simulink model "mpc_works"  (R2019b)
settings: Solver=VariableStepAuto  StartTime=0.0  StopTime=100  RelTol=1e-3
values from neighbouring files (symbols this model uses):
  Ts = 0.1    [mpcobj1.m]
libraries: simulink x1, mpclib x1
settings Model: PacingRate=0.350000  Creator=deepa  LastModifiedBy=deepa
settings SolverCC: MaxConsecutiveMinStep=100

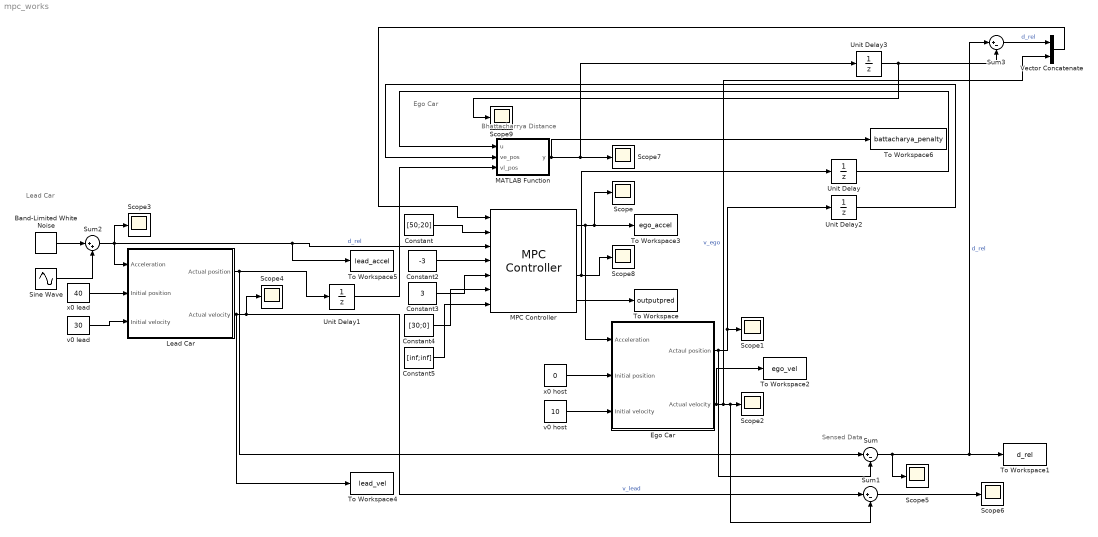
== system mpc_works ==
  note: Bhattacharrya Distance
  note: Lead Car
  note: Sensed Data
  note: Ego Car
  Band-Limited White Noise : simulink/Sources/Band-Limited White Noise  Cov=0.1  Ts=0.1  seed=[23341]
  Constant : Constant  Value=[50;20]
  Constant2 : Constant  Value=-3
  Constant3 : Constant  Value=3
  Constant4 : Constant  Value=[30;0]
  Constant5 : Constant  Value=[inf;inf]
  Ego Car : Subsystem
  Lead Car : Subsystem
  MATLAB Function : MATLAB Function  TreatAsAtomicUnit=on
  MPC Controller : mpclib/MPC Controller  SCDEnableBlockLinearizationSpecification=on  mpcobj=mpcobj  is_multiple=0  enable_value=0  return_u0=off  updateMPCinCallerWorkspace=on  md_inport=on  mv_inport=off  uref_inport=off  return_cost=off  return_mvseq=on  return_qpstatus=off  return_xseq=on  return_state=off  return_ovseq=on  state_inport=off  umin_inport=on  umax_inport=on  ymin_inport=on  ymax_inport=on  cc_inport=off  ywt_inport=off  uwt_inport=off  duwt_inport=off  rhoeps_inport=off  pm_inport=off  MaximumP=10  HorizonChoice=FixedHorizon  n_ts=0.1  n_p=10  n_mv=1  n_md=1  n_ud=0  n_mo=2  n_uo=0  BlockDataType=double  SampleTimeInherited=off  switch_inport=off
  Scope{,1..9} (10 alike) : Scope
  Sine Wave : Sin  Frequency=0.5  SampleTime=Ts
  Sum : Sum  Inputs=|+-
  Sum1 : Sum  Inputs=|+-
  Sum2 : Sum  Inputs=|++
  Sum3 : Sum  Inputs=|+-
  To Workspace : ToWorkspace  VariableName=outputpred  SampleTime=-1
  To Workspace1 : ToWorkspace  VariableName=d_rel  SaveFormat=Timeseries  SampleTime=-1
  To Workspace2 : ToWorkspace  VariableName=ego_vel  SaveFormat=Timeseries  SampleTime=-1
  To Workspace3 : ToWorkspace  VariableName=ego_accel  SaveFormat=Timeseries  SampleTime=-1
  To Workspace4 : ToWorkspace  VariableName=lead_vel  SaveFormat=Timeseries  SampleTime=-1
  To Workspace5 : ToWorkspace  VariableName=lead_accel  SaveFormat=Timeseries  SampleTime=-1
  To Workspace6 : ToWorkspace  VariableName=battacharya_penalty  SaveFormat=Timeseries  SampleTime=-1
  Unit Delay : UnitDelay  InitialCondition=rand(11,4)  SampleTime=-1  HasFrameUpgradeWarning=on
  Unit Delay1 : UnitDelay  SampleTime=-1  HasFrameUpgradeWarning=on
  Unit Delay2 : UnitDelay  SampleTime=-1  HasFrameUpgradeWarning=on
  Unit Delay3 : UnitDelay  SampleTime=-1  HasFrameUpgradeWarning=on
  Vector Concatenate : Concatenate
  v0 host : Constant  Value=10  SampleTime=Ts
  v0 lead : Constant  Value=30  SampleTime=Ts
  x0 host : Constant  Value=0  SampleTime=Ts
  x0 lead : Constant  Value=40  SampleTime=Ts
  wires:
  Sum2/1 -> MPC Controller/3, To Workspace5/1, Scope3/1, Lead Car/1(Acceleration)  "d_rel"
  Lead Car/1(Actual position) -> Unit Delay1/1, Sum/1
  Lead Car/2(Actual velocity) -> Scope4/1, Sum1/1, To Workspace4/1  "v_lead"
  Band-Limited White Noise/1 -> Sum2/1
  v0 lead/1 -> Lead Car/3(Initial velocity)
  x0 lead/1 -> Lead Car/2(Initial position)
  Sum/1 -> Sum3/1, To Workspace1/1, Scope5/1  "d_rel"
  Sum1/1 -> Scope6/1
  MPC Controller/3 -> Unit Delay/1, Scope8/1
  Sine Wave/1 -> Sum2/2
  x0 host/1 -> Ego Car/2(Initial position)
  Constant2/1 -> MPC Controller/4
  Constant3/1 -> MPC Controller/5
  Unit Delay3/1 -> Scope9/1, Sum3/2
  Constant4/1 -> MPC Controller/6
  Constant/1 -> MPC Controller/2
  MATLAB Function/1(y) -> Unit Delay3/1, Scope7/1, To Workspace6/1
  v0 host/1 -> Ego Car/3(Initial velocity)
  Vector Concatenate/1 -> MPC Controller/1
  Constant5/1 -> MPC Controller/7
  Sum3/1 -> Vector Concatenate/1  "d_rel"
  Ego Car/2(Actual velocity) -> Sum1/2, Scope2/1, Vector Concatenate/2, To Workspace2/1  "v_ego"
  Unit Delay/1 -> MATLAB Function/1(u)
  Unit Delay2/1 -> MATLAB Function/2(ve_pos)
  MPC Controller/4 -> To Workspace/1
  Ego Car/1(Actaul position) -> Unit Delay2/1, Scope1/1, Sum/2
  MPC Controller/1 -> To Workspace3/1, Scope/1, Ego Car/1(Acceleration)
  Unit Delay1/1 -> MATLAB Function/3(vl_pos)

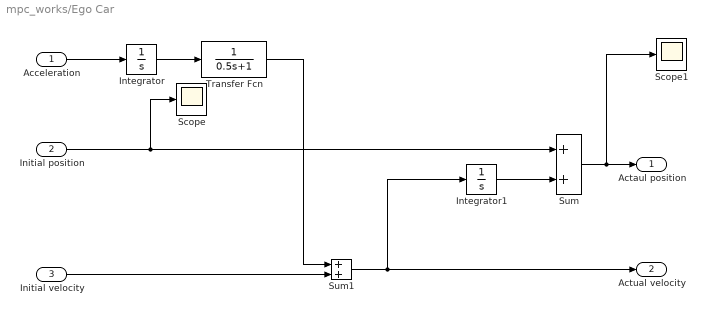
== system mpc_works/Ego Car ==
  Acceleration : Inport
  Initial position : Inport  Port=2
  Initial velocity : Inport  Port=3
  Integrator : Integrator
  Integrator1 : Integrator
  Scope : Scope
  Scope1 : Scope
  Sum : Sum
  Sum1 : Sum
  Transfer Fcn : TransferFcn  Denominator=[0.5 1]
  Actaul position : Outport  VectorParamsAs1DForOutWhenUnconnected=off
  Actual velocity : Outport  Port=2  VectorParamsAs1DForOutWhenUnconnected=off
  wires:
  Sum1/1 -> Integrator1/1, Actual velocity/1
  Initial velocity/1 -> Sum1/2
  Sum/1 -> Scope1/1, Actaul position/1
  Transfer Fcn/1 -> Sum1/1
  Integrator/1 -> Transfer Fcn/1
  Acceleration/1 -> Integrator/1
  Initial position/1 -> Scope/1, Sum/1
  Integrator1/1 -> Sum/2

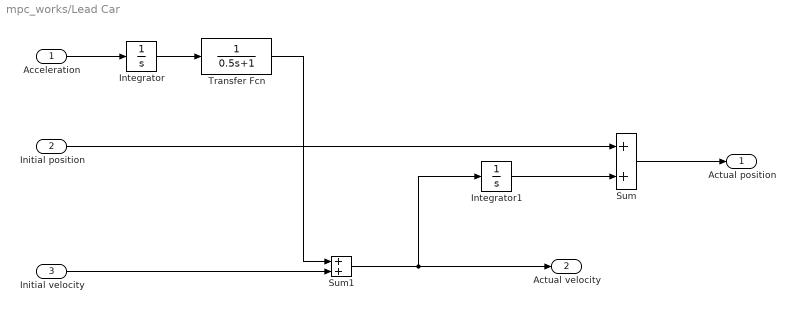
== system mpc_works/Lead Car ==
  Acceleration : Inport
  Initial position : Inport  Port=2
  Initial velocity : Inport  Port=3
  Integrator : Integrator
  Integrator1 : Integrator
  Sum : Sum
  Sum1 : Sum
  Transfer Fcn : TransferFcn  Denominator=[0.5 1]
  Actual position : Outport  VectorParamsAs1DForOutWhenUnconnected=off
  Actual velocity : Outport  Port=2  VectorParamsAs1DForOutWhenUnconnected=off
  wires:
  Transfer Fcn/1 -> Sum1/1
  Initial velocity/1 -> Sum1/2
  Sum/1 -> Actual position/1
  Integrator/1 -> Transfer Fcn/1
  Sum1/1 -> Integrator1/1, Actual velocity/1
  Acceleration/1 -> Integrator/1
  Initial position/1 -> Sum/1
  Integrator1/1 -> Sum/2

== matlab function mpc_works/MATLAB Function ==
  data: u input; y output; ve_pos input; vl_pos input
function y = fcn(u,ve_pos,vl_pos)
vl = u(:,2);
ve = u(:,3);
ve_ref = vl(1);
vl_pos = vl_pos+0.1*vl;
ve_pos = ve_pos+0.1*ve;
vl_var = var(vl_pos);
ve_var = var(ve_pos);
vl_mean = mean(vl_pos);
ve_mean = mean(ve_pos);
a = vl_var^2/ve_var^2;
b = ve_var^2/vl_var^2;
c = a+b+2;
d = (ve_mean-vl_mean)^2;
e = ve_var^2 + vl_var^2;
f = d/e;
g = 0.25*c;
h = 0.25*f;
%Bdist = 0.25*log(g)+h;
if vl_var<-0.00001||ve_var<-0.00001
    Bdist = 0.25*d;
else
    Bdist = 0.25*log(g)+h;
end

%Bdist = Bdist/90;-----------Bdist/10^9
thresBd = (1 - 1/(1+exp(-Bdist/10^7)))*10;
% if thresBd<2
%     output = 5;
% else
%     output = 0;
% end

y = thresBd;
